simulink model "issue_model_2093701"  (Simulink 9.2)
settings: Solver=VariableStepAuto  StartTime=0.0  StopTime=0.0  RelTol=1e-3
settings Model: Creator=ksurende  LastModifiedBy=汪海博
settings DataIOCC: LimitDataPoints=off  SaveFormat=Dataset  SignalLoggingSaveFormat=Dataset
settings DebuggingCC: UnderspecifiedInitializationDetection=Simplified  MergeDetectMultiDrivingBlocksExec=error  FcnCallInpInsideContextMsg=error  StateNameClashWarn=none  SFUnexpectedBacktrackingDiag=error  SFNoUnconditionalDefaultTransitionDiag=error  SFExecutionAtInitializationDiag=warning
settings HardwareCC: ProdBitPerPointer=64  ProdBitPerSizeT=64  ProdBitPerPtrDiffT=64  ProdLargestAtomicFloat=Float  ProdIntDivRoundTo=Zero  ProdEndianess=LittleEndian  ProdWordSize=64  ProdHWDeviceType=Intel->x86-64 (Windows64)
settings ModelReferenceCC: PropagateSignalLabelsOutOfModel=on
settings GRTTargetCC: TargetLangStandard=C99 (ISO)  GeneratePreprocessorConditionals=Use local settings  CombineOutputUpdateFcns=on  GRTInterface=off
settings ConfigComp: CovMetricSettings=dwe  CovHtmlReporting=off  CovSaveCumulativeToWorkspaceVar=off  CovSaveSingleToWorkspaceVar=off  CovExternalEMLEnable=on

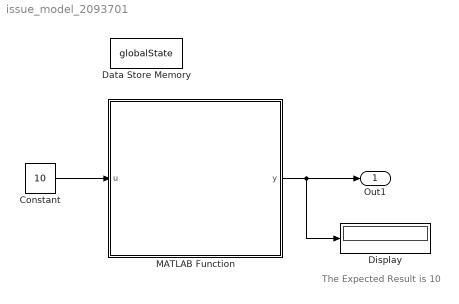
== system issue_model_2093701 ==
  note: The Expected Result is 10
  Constant : Constant  Value=10
  Data Store Memory : DataStoreMemory  DataStoreName=globalState  ReadBeforeWriteMsg=warning  WriteAfterWriteMsg=warning  WriteAfterReadMsg=warning  ShowAdditionalParam=off  OutDataTypeStr=double  Dimensions=1
  Display : Display
  MATLAB Function : MATLAB Function  TreatAsAtomicUnit=on
  Out1 : Outport
  wires:
  MATLAB Function/1(y) -> Display/1, Out1/1
  Constant/1 -> MATLAB Function/1(u)

== matlab function MATLAB Function ==
  data: u input double; y output double; globalState data_store_memory double
function y = fcn(u)

y = issue_example(u);
end

function out = issue_example(idx)
    global globalState;
    globalState = 0;

    while(globalState < idx  && ...
          updateGlobalState())
    end 

    out = globalState;
end 

function out = updateGlobalState()
    coder.inline('never');
    global globalState;
    globalState = globalState + 1;

    if(globalState > 100)
        out = false;
        return;
    end
    out = true;
end
